simulink model "problem1"  (R2020b)
settings: Solver=VariableStepAuto  StartTime=0.0  StopTime=10.0  RelTol=1e-3
undefined symbols (not defined in the file): b, K1, K12, M1, M2
settings Model: Creator=sonal  LastModifiedBy=sonal

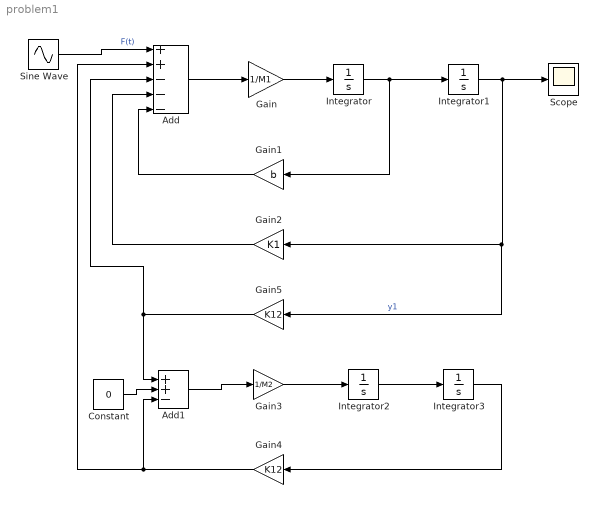
== system problem1 ==
  Add : Sum  Inputs=++---
  Add1 : Sum  Inputs=++-
  Constant : Constant  Value=0
  Gain : Gain  Gain=1/M1
  Gain1 : Gain  Gain=b
  Gain2 : Gain  Gain=K1
  Gain3 : Gain  Gain=1/M2
  Gain4 : Gain  Gain=K12
  Gain5 : Gain  Gain=K12
  Integrator{,1..3} (4 alike) : Integrator
  Scope : Scope
  Sine Wave : Sin  Amplitude=2  Frequency=10  SampleTime=0
  wires:
  Add/1 -> Gain/1
  Gain3/1 -> Integrator2/1
  Gain4/1 -> Add1/3, Add/2
  Add1/1 -> Gain3/1
  Gain1/1 -> Add/5
  Integrator1/1 -> Scope/1, Gain5/1, Gain2/1  "y1"
  Gain5/1 -> Add1/1, Add/3
  Integrator/1 -> Gain1/1, Integrator1/1
  Integrator2/1 -> Integrator3/1
  Gain2/1 -> Add/4
  Integrator3/1 -> Gain4/1
  Constant/1 -> Add1/2
  Gain/1 -> Integrator/1
  Sine Wave/1 -> Add/1  "F(t)"
